simulink model "out_model"  (R2024a)
settings: Solver=VariableStepAuto  StartTime=0.0  StopTime=6  FixedStep=0.0001  RelTol=1e-7  AbsTol=1e-8
values from neighbouring files (symbols this model uses):
  A = [11 -2 13; 6 -1 6; -6 -1 -8]    [comp_sost.m]    (also in meandr.m = [0 1; 0 0]; out.m; out_copy.m; rank_extended.m)
  B = [2; 0; 0]    [comp_sost.m]    (also in meandr.m = [0; 1]; out.m; out_copy.m; slezh_sost.m)
  Bf = [-6 0 0 -1; 0 0 0 0; 6 0 0 0]    [comp_sost.m]    (also in out.m; out_copy.m; rank_extended.m)
  C = [1 0]    [meandr.m]    (also in out.m = [2 -2 1]; out_copy.m = [2 -2 1]; rank_extended.m = [2 -2 1])
  Cz = [-2 3 -1]    [comp_sost.m]    (also in meandr.m = -C; out.m; out_copy.m = C; slezh_sost.m)
  D = [1 2 1 -1]    [out.m]    (also in out_copy.m; rank_extended.m)
  Dz = 16/pi * [1 0 1/3 0 1/5 0]    [meandr.m]    (also in out.m = [3 4 2 -3]; out_copy.m = D; slezh_sost.m = [3 4 2 -3])
  G = [35 56 22 -42; -11 -17 -7 12; -6 -10 -5 10; 11 18 6 -13]    [comp_sost.m]    (also in meandr.m = [0 1 0 0 0 0; -1 0 0 0 0 0; 0 0 0 3 0 0; 0 0 -3 0 0 0; 0 0 0; out.m; out_copy.m; rank_extended.m)
  K1 = -inv(R)*B'*P    [comp_sost.m]    (also in meandr.m; out.m = -R\B'*P; out_copy.m; slezh_sost.m)
  K2 = double(Y_sol - K1*P_sol)    [comp_sost.m]    (also in meandr.m; out.m; out_copy.m; slezh_sost.m)
  L1 = L(1:3, :)    [out.m]    (also in out_copy.m)
  L2 = L(4:7, :)    [out.m]    (also in out_copy.m)
settings Model: Creator=ventus  LastModifiedBy=ventus

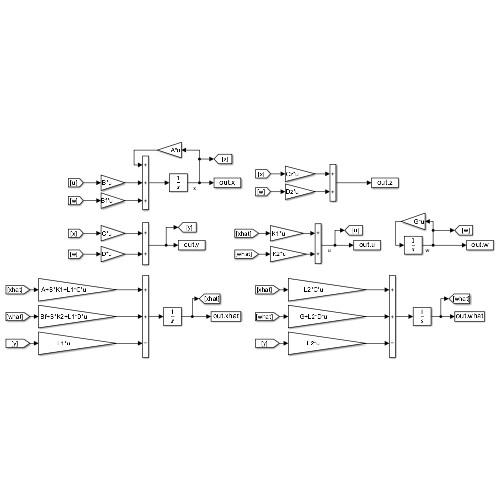
[thumbnail: Simulink's stored preview of the top-level diagram]
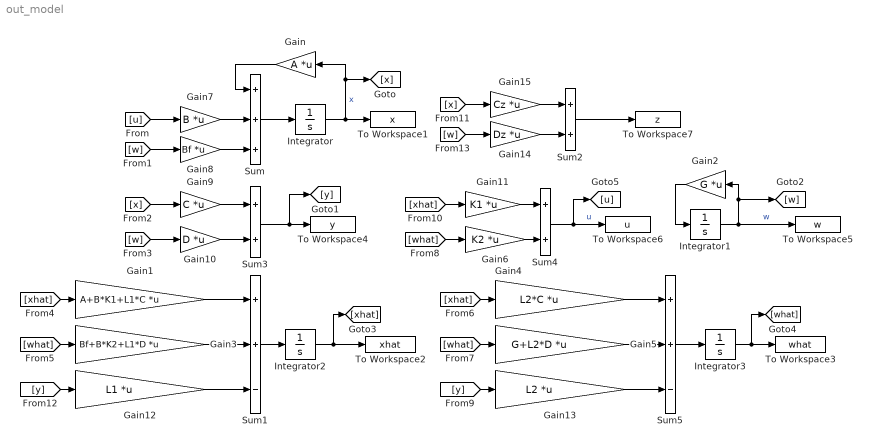
== system out_model ==
  Gain : Gain  Gain=A  Multiplication=Matrix(K*u)
  Gain1 : Gain  Gain=A+B*K1+L1*C  Multiplication=Matrix(K*u)
  Gain10 : Gain  Gain=D  Multiplication=Matrix(K*u)
  Gain11 : Gain  Gain=K1  Multiplication=Matrix(K*u)
  Gain12 : Gain  Gain=L1  Multiplication=Matrix(K*u)
  Gain13 : Gain  Gain=L2  Multiplication=Matrix(K*u)
  Gain14 : Gain  Gain=Dz  Multiplication=Matrix(K*u)
  Gain15 : Gain  Gain=Cz  Multiplication=Matrix(K*u)
  Gain2 : Gain  Gain=G  Multiplication=Matrix(K*u)
  Gain3 : Gain  Gain=Bf+B*K2+L1*D  Multiplication=Matrix(K*u)
  Gain4 : Gain  Gain=L2*C  Multiplication=Matrix(K*u)
  Gain5 : Gain  Gain=G+L2*D  Multiplication=Matrix(K*u)
  Gain6 : Gain  Gain=K2  Multiplication=Matrix(K*u)
  Gain7 : Gain  Gain=B  Multiplication=Matrix(K*u)
  Gain8 : Gain  Gain=Bf  Multiplication=Matrix(K*u)
  Gain9 : Gain  Gain=C  Multiplication=Matrix(K*u)
  Integrator : Integrator  InitialCondition=[1; 1; 1]
  Integrator1 : Integrator  InitialCondition=[1; 1; 1; 1]
  Integrator2 : Integrator
  Integrator3 : Integrator
  Sum : Sum  Inputs=+++
  Sum1 : Sum  Inputs=++-
  Sum2 : Sum
  Sum3 : Sum
  Sum4 : Sum
  Sum5 : Sum  Inputs=++-
  To Workspace1 : ToWorkspace  VariableName=x  SaveFormat=Timeseries  SampleTime=-1
  To Workspace2 : ToWorkspace  VariableName=xhat  SaveFormat=Timeseries  SampleTime=-1
  To Workspace3 : ToWorkspace  VariableName=what  SaveFormat=Timeseries  SampleTime=-1
  To Workspace4 : ToWorkspace  VariableName=y  SaveFormat=Timeseries  SampleTime=-1
  To Workspace5 : ToWorkspace  VariableName=w  SaveFormat=Timeseries  SampleTime=-1
  To Workspace6 : ToWorkspace  VariableName=u  SaveFormat=Timeseries  SampleTime=-1
  To Workspace7 : ToWorkspace  VariableName=z  SaveFormat=Timeseries  SampleTime=-1
  wires:
  Sum/1 -> Integrator/1
  Integrator/1 -> To Workspace1/1, [x], Gain/1  "x"
  Gain/1 -> Sum/1
  Gain7/1 -> Sum/2
  [u] -> Gain7/1
  Gain8/1 -> Sum/3
  [w] -> Gain8/1
  [x] -> Gain9/1
  [w] -> Gain10/1
  Gain10/1 -> Sum3/2
  Gain9/1 -> Sum3/1
  Sum3/1 -> [y], To Workspace4/1
  Integrator1/1 -> Gain2/1, [w], To Workspace5/1  "w"
  Gain2/1 -> Integrator1/1
  [xhat] -> Gain1/1
  [what] -> Gain3/1
  Gain1/1 -> Sum1/1
  Gain3/1 -> Sum1/2
  Sum1/1 -> Integrator2/1
  Integrator2/1 -> To Workspace2/1, [xhat]
  [what] -> Gain5/1
  Gain5/1 -> Sum5/2
  Gain4/1 -> Sum5/1
  [xhat] -> Gain4/1
  Integrator3/1 -> To Workspace3/1, [what]
  Sum5/1 -> Integrator3/1
  [what] -> Gain6/1
  [xhat] -> Gain11/1
  Gain11/1 -> Sum4/1
  Gain6/1 -> Sum4/2
  [y] -> Gain12/1
  Gain12/1 -> Sum1/3
  [y] -> Gain13/1
  Gain13/1 -> Sum5/3
  Sum4/1 -> To Workspace6/1, [u]  "u"
  Gain14/1 -> Sum2/2
  Gain15/1 -> Sum2/1
  Sum2/1 -> To Workspace7/1
  [w] -> Gain14/1
  [x] -> Gain15/1
